simulink model "cw2sim"  (R2020b)
settings: Solver=VariableStepAuto  StartTime=0.0  StopTime=20  RelTol=1e-3
values from neighbouring files (symbols this model uses):
  k = 1    [cw2.m]
  k_ster = 2.3    [cw2.m]
  omega_0 = 2    [cw2.m]
  T = 2    [cw2.m]
  T_ster = 1    [cw2.m]
settings Model: Creator=pmiel  LastModifiedBy=stasz

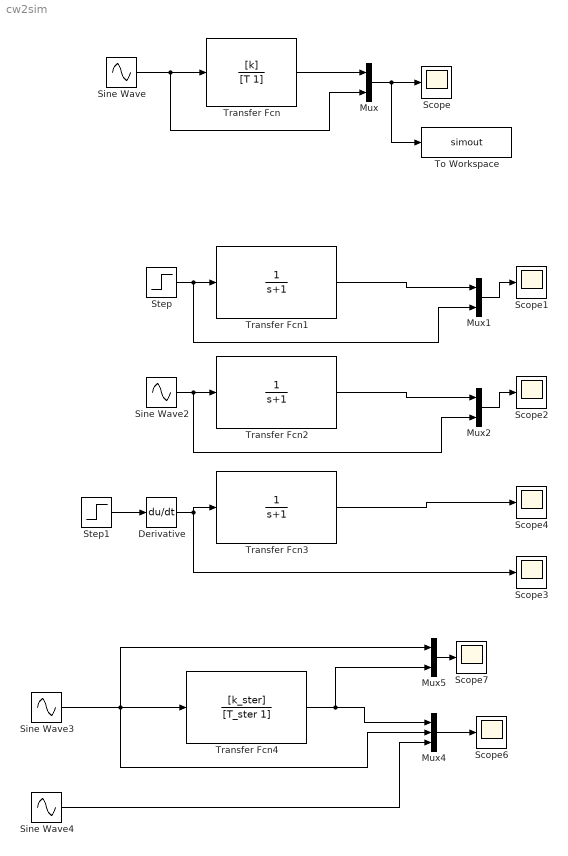
== system cw2sim ==
  Derivative : Derivative
  Mux{,1..2,5} (4 alike) : Mux  Inputs=2
  Mux4 : Mux  Inputs=3
  Scope{,1..4,6..7} (7 alike) : Scope
  Sine Wave : Sin  Frequency=omega_0  SampleTime=0
  Sine Wave2 : Sin  SampleTime=0
  Sine Wave3 : Sin  Frequency=omega_0  SampleTime=0
  Sine Wave4 : Sin  Frequency=omega_0  Phase=-1  SampleTime=0
  Step : Step  SampleTime=0
  Step1 : Step  SampleTime=0
  To Workspace : ToWorkspace  VariableName=simout  SaveFormat=Timeseries  SampleTime=-1
  Transfer Fcn : TransferFcn  Numerator=[k]  Denominator=[T 1]
  Transfer Fcn1 : TransferFcn  Denominator=[1 1]
  Transfer Fcn2 : TransferFcn  Denominator=[1 1]
  Transfer Fcn3 : TransferFcn  Denominator=[1 1]
  Transfer Fcn4 : TransferFcn  Numerator=[k_ster]  Denominator=[T_ster 1]
  wires:
  Mux/1 -> To Workspace/1, Scope/1
  Transfer Fcn/1 -> Mux/1
  Step/1 -> Mux1/2, Transfer Fcn1/1
  Mux1/1 -> Scope1/1
  Transfer Fcn1/1 -> Mux1/1
  Transfer Fcn2/1 -> Mux2/1
  Mux2/1 -> Scope2/1
  Sine Wave2/1 -> Mux2/2, Transfer Fcn2/1
  Transfer Fcn3/1 -> Scope4/1
  Derivative/1 -> Scope3/1, Transfer Fcn3/1
  Step1/1 -> Derivative/1
  Transfer Fcn4/1 -> Mux5/2, Mux4/1
  Sine Wave4/1 -> Mux4/3
  Sine Wave3/1 -> Mux5/1, Mux4/2, Transfer Fcn4/1
  Mux5/1 -> Scope7/1
  Mux4/1 -> Scope6/1
  Sine Wave/1 -> Transfer Fcn/1, Mux/2
